simulink model "MySusp_Stabi_RTW"  (R2022a)
settings: Solver=ode1  StartTime=0.0  StopTime=inf  FixedStep=0.001  RelTol=1e-3
PreLoadFcn:
  | vehicle = 'Car'; if ~length(which('cmself')), cmenv; end
  | MySusp_Stabi_RTW_bus
  | MySusp_Stabi_RTW_params
InitFcn:
  | vehicle = 'Car'; if ~length(which('cmself')), cmenv; end
  | MySusp_Stabi_RTW_bus
undefined symbols (not defined in the file or in its folder): Stiffness
Description:
  | CarMaker Plug-in Model Target
settings Model: ModifiedByFormat=IPG  Creator=IPG  LastModifiedBy=IPG
settings SolverCC: AlgebraicLoopSolver=TrustRegion
settings DataIOCC: ReturnWorkspaceOutputs=off
settings DebuggingCC: UnconnectedInputMsg=warning  UnconnectedOutputMsg=warning  UnconnectedLineMsg=warning  PregeneratedLibrarySubsystemCodeDiagnostic=none  SFMachineParentedDataDiag=warning  ArithmeticOperatorsInVariantConditions=warning
settings SFSimCC: SimUseLocalCustomCode=off  CustomCodeUndefinedFunction=UseInterfaceOnly
settings RTWCC: Description=CarMaker Plug-in Model Target  SystemTargetFile=CarMaker.tlc  TemplateMakefile=CarMaker_unix-win64.tmf  RTWUseLocalCustomCode=off  DLArmComputeVersion=19.05
settings CodeAppCC: MaxIdLength=127  StateflowObjectComments=on
settings STFCustomTargetCC: TargetLangStandard=C99 (ISO)  CombineOutputUpdateFcns=on  CodeInterfacePackaging=Reusable function  GRTInterface=off  GenerateAllocFcn=on  SystemTargetFile=CarMaker.tlc
settings GRTTargetCC: ParMdlRefBuildCompliant=off  CompOptLevelCompliant=off  ConcurrentExecutionCompliant=off  MatFileLogging=off  CodeInterfacePackaging=Reusable function  CPPClassGenCompliant=off  GenerateAllocFcn=on  UseToolchainInfoCompliant=off  RTWCAPISignals=on  RTWCAPIParams=on  RTWCAPIStates=on

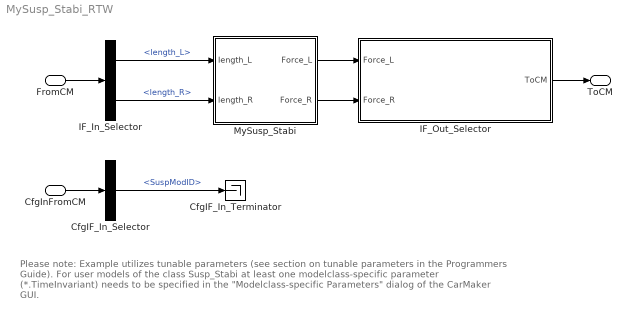
== system MySusp_Stabi_RTW ==
  note: Please note: Example utilizes tunable parameters (see section on tunable parameters in the Programmers Guide).
      |
      | For user models of the class Susp_Stabi at least one modelclass-specific parameter (*.TimeInvariant) needs to be specified in the
      | "Modelclass-specific Parameters" dialog of the CarMaker GUI.
  FromCM : Inport  OutDataTypeStr=Bus: cmSusp_StabiIn
  CfgInFromCM : Inport  Port=2  OutDataTypeStr=Bus: cmSusp_StabiCfgIn
  CfgIF_In_Selector : BusSelector  OutputSignals=SuspModID
  CfgIF_In_Terminator : Terminator
  IF_In_Selector : BusSelector  OutputSignals=length_L,length_R
  IF_Out_Selector : Subsystem  mask(Signal Selection){}
      mask help: Signal Selection Block
      settings: OpenFcn=cmSignalSelect('SignalSelection_CB',gcb)
  MySusp_Stabi : Subsystem
  ToCM : Outport  OutDataTypeStr=Bus: cmSusp_StabiOut  VectorParamsAs1DForOutWhenUnconnected=off
  wires:
  FromCM/1 -> IF_In_Selector/1
  IF_Out_Selector/1(ToCM) -> ToCM/1
  CfgInFromCM/1 -> CfgIF_In_Selector/1
  CfgIF_In_Selector/1 -> CfgIF_In_Terminator/1  "<SuspModID>"
  IF_In_Selector/1 -> MySusp_Stabi/1(Iength_L)  "<length_L>"
  IF_In_Selector/2 -> MySusp_Stabi/2(length_R)  "<length_R>"
  MySusp_Stabi/1(Force_L) -> IF_Out_Selector/1(Force_L)
  MySusp_Stabi/2(Force_R) -> IF_Out_Selector/2(Force_R)

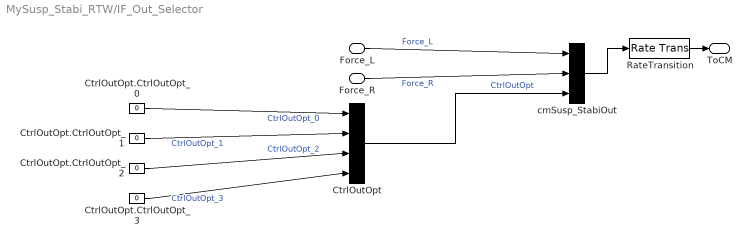
== system MySusp_Stabi_RTW/IF_Out_Selector ==
  Force_L : Inport
  Force_R : Inport  Port=2
  CtrlOutOpt : BusCreator  Inputs=4
  CtrlOutOpt.CtrlOutOpt_{0..3} (4 alike) : Constant  Value=0
  RateTransition : RateTransition  OutPortSampleTime=str2num(get_param(bdroot,'FixedStep'))
  cmSusp_StabiOut : BusCreator  Inputs=3
  ToCM : Outport
  wires:
  RateTransition/1 -> ToCM/1
  cmSusp_StabiOut/1 -> RateTransition/1
  CtrlOutOpt/1 -> cmSusp_StabiOut/3  "CtrlOutOpt"
  CtrlOutOpt.CtrlOutOpt_0/1 -> CtrlOutOpt/1  "CtrlOutOpt_0"
  CtrlOutOpt.CtrlOutOpt_1/1 -> CtrlOutOpt/2  "CtrlOutOpt_1"
  CtrlOutOpt.CtrlOutOpt_2/1 -> CtrlOutOpt/3  "CtrlOutOpt_2"
  CtrlOutOpt.CtrlOutOpt_3/1 -> CtrlOutOpt/4  "CtrlOutOpt_3"
  Force_L/1 -> cmSusp_StabiOut/1  "Force_L"
  Force_R/1 -> cmSusp_StabiOut/2  "Force_R"

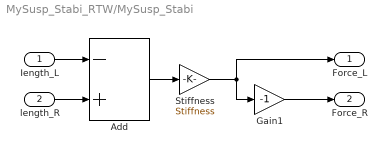
== system MySusp_Stabi_RTW/MySusp_Stabi ==
  Iength_L : Inport
  length_R : Inport  Port=2
  Add : Sum  Inputs=-+
  Gain1 : Gain  Gain=-1
  Stiffness : Gain  Gain=Stiffness
  Force_L : Outport  VectorParamsAs1DForOutWhenUnconnected=off
  Force_R : Outport  Port=2  VectorParamsAs1DForOutWhenUnconnected=off
  wires:
  Stiffness/1 -> Force_L/1, Gain1/1
  Gain1/1 -> Force_R/1
  Iength_L/1 -> Add/1
  length_R/1 -> Add/2
  Add/1 -> Stiffness/1
